simulink model "Frequency_scanning_2024a"  (R2024a)
settings: Solver=FixedStepAuto  StartTime=0  StopTime=2  FixedStep=Ts  RelTol=1e-3
InitFcn:
  | load('myData.mat')
  | 
  | %% Define parameters
  | xi=0;
  | w = 2*pi*50;
  | ApparatusPowerFlow{2} = [-P,-Q,V0,xi,w];
  | 
  | %% Mode
  | ApparatusType{2} = 10;
values from neighbouring files (symbols this model uses):
  x_e = [i_d; i_q; i_d_i; i_q_i; v_d_i; v_q_i; theta; v_dc; v_dc_i; i; i_i; v_lk; p_sum_i; p_lk_i]    [InterlinkAcDcB2B.m]
undefined symbols (not defined in the file or in its folder): ApparatusDiscreDamping, ApparatusPara, ApparatusPowerFlow, ApparatusType, cycles_n, DiscIntNeverNeededParam, f_end, f_start, harmonics_deg, n_sample, OtherInputs, PowerFlow, settle_time, start_time, submag, supmag, Ts, Vbase, Wbase, Zbase
libraries: SimplusGT x4, spsGroundLib x3, simulink x3, spsControlledVoltageSourceLib x3, spsVoltageMeasurementLib x1, spsThreePhaseSeriesRLCBranchLib x1, spspowerguiLib x1
settings Model: Creator=Yuming  LastModifiedBy=Yuming
settings DataIOCC: SaveOutput=off  SignalLogging=off  DSMLogging=off  InspectSignalLogs=on  SaveTime=off  ReturnWorkspaceOutputs=off
settings ConfigComp: CovBoundaryAbsTol=1.0e-5

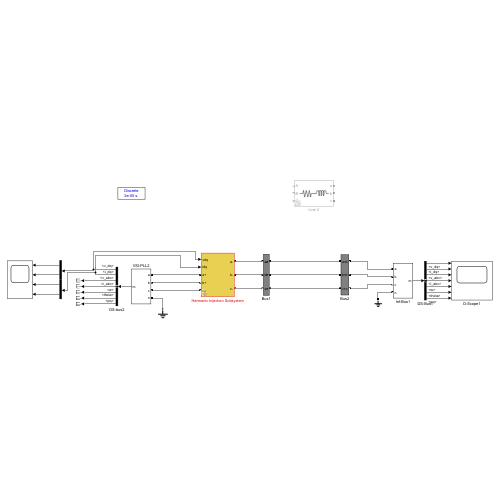
[thumbnail: Simulink's stored preview of the top-level diagram]
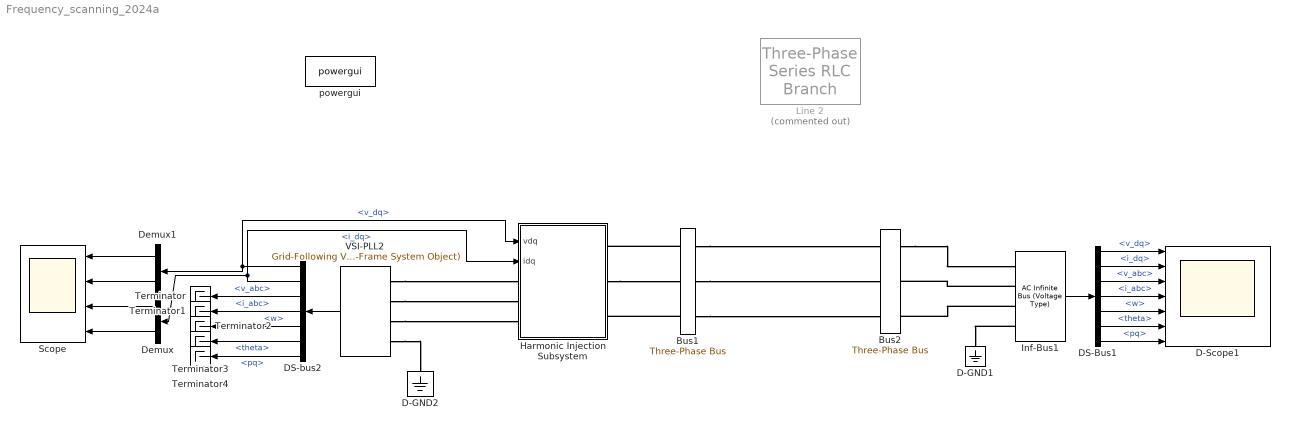
== system Frequency_scanning_2024a ==
  Bus1 : SimplusGT/Three-Phase Bus  Vbase=1  Sbase=1
      settings: SourceProductName=Simplus Grid Tool
  Bus2 : SimplusGT/Three-Phase Bus  Vbase=1  Sbase=1
      settings: SourceProductName=Simplus Grid Tool
  D-GND1 : spsGroundLib/Ground  LConnTagsString=a
  D-GND2 : spsGroundLib/Ground  LConnTagsString=a
  D-Scope1 : Scope  NumInputPorts=7
  DS-Bus1 : BusSelector  OutputSignals=v_dq,i_dq,v_abc,i_abc,w,theta,pq
  DS-bus2 : BusSelector  OutputSignals=v_dq,i_dq,v_abc,i_abc,w,theta,pq
  Demux : Demux  Outputs=2
  Demux1 : Demux  Outputs=2
  Harmonic Injection Subsystem : Subsystem  mask{f_start=f_start, f_end=f_end, n_pts=n_sample, cycle_collected=cycles_n, fundal_freq=50, start_time=start_time, settling_time=settle_time, subsyc_mag=submag, supsyc_mag=supmag, initial_phase=0, phase_angle=harmonics_deg}
      mask prompts: f_start "Start frequency (Hz)"; f_end "End frequency (Hz)"; n_pts "Number of samples"; cycle_collected "Full cycles in window"; fundal_freq "Fundamental Frequency (Hz)"; start_time "Start Time (sec)"; settling_time "Pre-settling duration (sec)"; subsyc_mag "Sub-synchronous magnitude (pu)"; supsyc_mag "Super-synchronous magnitude (pu)"; initial_phase "Initial phase (rad)"; phase_angle "Initial phase angle (w.r.t. fundamental) [deg]"
      mask init:
      | % Mask Initialization Code
      | freq_list = logspace(log10(f_start), log10(f_end), n_pts).';
      | idx_list  = (1:n_pts).';
      mask DialogControl DescGroupVar Prompt: Harmonic signal generator
      mask DialogControl DescTextVar Prompt: This block implements a harmonic signal generator.   It produces a fundamental component at the specified fundamental frequency,   together with two symmetrical sidebands (sub-synchronous and super-synchronous)   around the fundamental.
  Inf-Bus1 : SimplusGT/AC Infinite Bus (Voltage Type)  Ts=Ts  Sbase=Sbase  Vbase=Vbase  Wbase=Wbase  vd=PowerFlow{1}(3)  vq=0  theta0=PowerFlow{1}(4)  w=Wbase  R=1e-30
      settings: SourceProductName=Simplus Grid Tool
  Line 2 : spsThreePhaseSeriesRLCBranchLib/Three-Phase Series RLC Branch  Commented=on  LConnTagsString=A|B|C  RConnTagsString=A|B|C  BranchType=RL  Resistance=0.06*Zbase  Inductance=0.3*Zbase/Wbase  Capacitance=1e-6  Measurements=None
  Scope : Scope  NumInputPorts=4
  Terminator{,1..4} (5 alike) : Terminator
  VSI-PLL2 : SimplusGT/Grid-Following Voltage-Source Inverter (dq-Frame System Object)  Ts=Ts  Sbase=Sbase  Vbase=Vbase  Wbase=Wbase  ApparatusType=ApparatusType{2}  ApparatusPara=ApparatusPara{2}  PowerFlow=ApparatusPowerFlow{2}  x0=x_e{2}  OtherInputs=OtherInputs{2}  DiscreMethod=Hybrid Trapezoidal  EnableInsideModification=off  DiscreDampingFlag=on  DiscreDampingValue=ApparatusDiscreDamping{2}  LinearizationTimes=1  DirectFeedthrough=off
      settings: SourceProductName=Simplus Grid Tool
  powergui : spspowerguiLib/powergui  Priority=1  SimulationMode=Discrete  SampleTime=Ts  frequency=60  Iterations=50  frequencyindice=0  Pbase=100e6  ErrMax=1e-4  UnitsV=kV  UnitsW=MW  buscounter=0  FunctionMessages=off  echomessages=off  EnableUseOfTLC=off  CurrentSourceSwitches=off  DisableSnubberDevices=off  DisableRonSwitches=off  DisableVfSwitches=off  DisplayEquations=off  AutomaticDiscreteSolvers=off  SolverType=Tustin/Backward Euler (TBE)  Interpol=off  ExternalGateDelay=off  methode=off  Ts=100  x0status=blocks  SPID=on  SwTol=0  HookPort=off  NonlinearTolerance=1e-4  nMaxIteration=100  ContinueOnMaxIteration=off  RestoreLinks=warning  ResistiveCurrentMeasurement=off  Frange=[0:2:500]  Ylog=off  Xlog=on  ShowGrid=off  save=off  variable=ZData  structure=0  ZoomFFT=off  StartTime=0.0  cycles=1  DisplayStyle=1  fundamental=60  FreqAxis=off  MaxFrequency=1000  frequencyindicesteady=1  RmsSteady=1  display=off
  wires:
  Inf-Bus1/1 -> DS-Bus1/1
  DS-Bus1/1 -> D-Scope1/1  "<v_dq>"
  DS-Bus1/2 -> D-Scope1/2  "<i_dq>"
  DS-Bus1/3 -> D-Scope1/3  "<v_abc>"
  DS-Bus1/4 -> D-Scope1/4  "<i_abc>"
  DS-Bus1/5 -> D-Scope1/5  "<w>"
  DS-Bus1/6 -> D-Scope1/6  "<theta>"
  DS-Bus1/7 -> D-Scope1/7  "<pq>"
  VSI-PLL2/1 -> DS-bus2/1
  DS-bus2/1 -> Demux1/1, Harmonic Injection Subsystem/1(vdq)  "<v_dq>"
  DS-bus2/2 -> Demux/1, Harmonic Injection Subsystem/2(idq)  "<i_dq>"
  DS-bus2/3 -> Terminator/1  "<v_abc>"
  DS-bus2/4 -> Terminator1/1  "<i_abc>"
  DS-bus2/5 -> Terminator2/1  "<w>"
  DS-bus2/6 -> Terminator3/1  "<theta>"
  DS-bus2/7 -> Terminator4/1  "<pq>"
  Demux1/1 -> Scope/1
  Demux1/2 -> Scope/2
  Demux/1 -> Scope/3
  Demux/2 -> Scope/4
  connections:
  Inf-Bus1/LConn4 -- D-GND1/LConn1
  VSI-PLL2/LConn4 -- D-GND2/LConn1
  Inf-Bus1/LConn2 -- Bus2/RConn2
  Inf-Bus1/LConn3 -- Bus2/RConn3
  Bus1/RConn2 -- Bus2/LConn2
  Bus1/RConn1 -- Bus2/LConn1
  Bus1/RConn3 -- Bus2/LConn3
  Bus2/RConn1 -- Inf-Bus1/LConn1
  Bus1/LConn1 -- Harmonic Injection Subsystem/RConn1
  Harmonic Injection Subsystem/RConn2 -- Bus1/LConn2
  Bus1/LConn3 -- Harmonic Injection Subsystem/RConn3
  VSI-PLL2/LConn1 -- Harmonic Injection Subsystem/LConn1
  VSI-PLL2/LConn2 -- Harmonic Injection Subsystem/LConn2
  VSI-PLL2/LConn3 -- Harmonic Injection Subsystem/LConn3

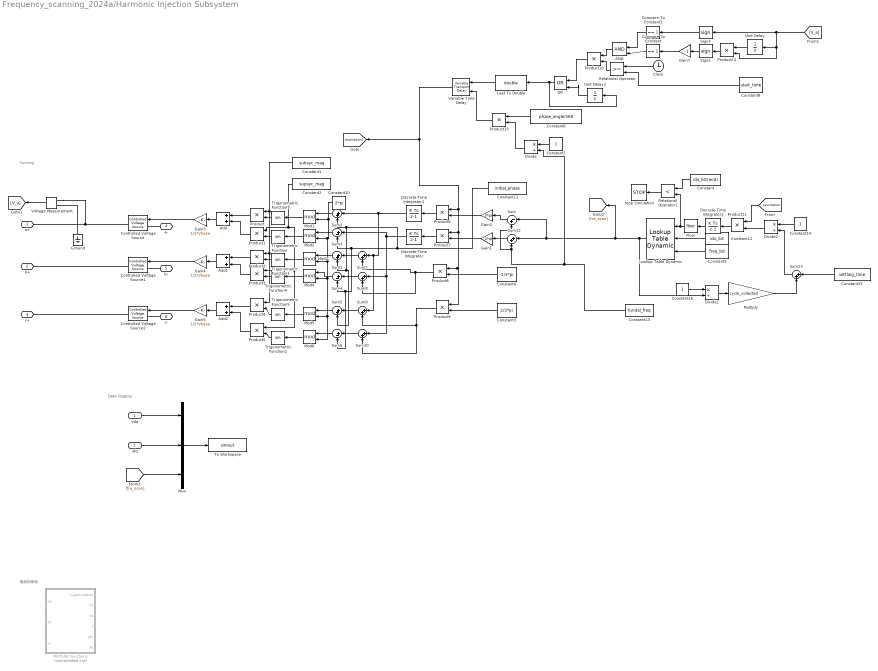
== system Frequency_scanning_2024a/Harmonic Injection Subsystem ==
  note: Data logging
  note: Yuming
  note: 废品回收站
  vdq : Inport
  idq : Inport  Port=2
  AND : Logic  IconShape=distinctive  AllPortsSameDT=off  OutDataTypeStr=boolean
  Add : Sum
  Add1 : Sum
  Add2 : Sum
  Cast To Double : DataTypeConversion  OutDataTypeStr=double  SaturateOnIntegerOverflow=off  RndMeth=Floor
  Clock : Clock
  Compare To Constant : simulink/Logic and Bit Operations/Compare To Constant  relop===  const=1  OutDataTypeStr=boolean
  Compare To Constant1 : simulink/Logic and Bit Operations/Compare To Constant  relop===  const=1  OutDataTypeStr=boolean
  Constant : Constant  Value=idx_list(end)
  Constant1 : Constant  Value=subsyc_mag
  Constant10 : Constant  Value=2*pi
  Constant11 : Constant  Value=initial_phase
  Constant12 : Constant  Value=idx_list
  Constant13 : Constant  Value=fundal_freq
  Constant14 : Constant
  Constant15 : Constant  Value=settling_time
  Constant16 : Constant
  Constant2 : Constant  Value=supsyc_mag
  Constant3 : Constant  Value=2/3*pi
  Constant4 : Constant  Value=-2/3*pi
  Constant5 : Constant  Value=freq_list
  Constant6 : Constant  Value=phase_angle/360
  Constant7 : Constant
  Constant9 : Constant  Value=start_time
  Controlled Voltage Source : spsControlledVoltageSourceLib/Controlled Voltage Source  Initialize=on  Source_Type=AC  Amplitude=0  Phase=0  Frequency=0  Measurements=None
  Controlled Voltage Source1 : spsControlledVoltageSourceLib/Controlled Voltage Source  Initialize=on  Source_Type=AC  Amplitude=0  Phase=0  Frequency=0  Measurements=None
  Controlled Voltage Source2 : spsControlledVoltageSourceLib/Controlled Voltage Source  Initialize=on  Source_Type=AC  Amplitude=0  Phase=0  Frequency=0  Measurements=None
  Discrete-Time Integrator : DiscreteIntegrator  SampleTime=Ts  ICPrevOutput=DiscIntNeverNeededParam  ICPrevScaledInput=DiscIntNeverNeededParam
  Discrete-Time Integrator1 : DiscreteIntegrator  SampleTime=Ts  ICPrevOutput=DiscIntNeverNeededParam  ICPrevScaledInput=DiscIntNeverNeededParam
  Discrete-Time Integrator2 : DiscreteIntegrator  SampleTime=-1  ICPrevOutput=DiscIntNeverNeededParam  ICPrevScaledInput=DiscIntNeverNeededParam
  Divide : Product  Inputs=*/
  Divide1 : Product  Inputs=*/
  Divide2 : Product  Inputs=*/
  Floor : Rounding
  Gain1 : Gain  Gain=2*pi
  Gain2 : Gain  Gain=2*pi
  Gain3 : Gain  Gain=1/2*Vbase
  Gain4 : Gain  Gain=1/2*Vbase
  Gain5 : Gain  Gain=1/2*Vbase
  Gain7 : Gain  Gain=-1
  Ground : spsGroundLib/Ground  LConnTagsString=a
  Lookup Table Dynamic : simulink/Lookup Tables/Lookup Table Dynamic  LookUpMeth=Interpolation-Use End Values  OutDataType=fixdt('double')  OutScaling=[]  OutputDataTypeScalingMode=Specify via dialog  OutDataTypeStr=double  DoSatur=off
  MATLAB Function1 : MATLAB Function  Commented=on  TreatAsAtomicUnit=on
  Mod{1..6} (6 alike) : Math  Operator=mod
  Multiply : Gain  Gain=cycle_collected
  Mux : Mux  Inputs=3
  OR : Logic  Operator=OR  IconShape=distinctive  AllPortsSameDT=off  OutDataTypeStr=boolean
  Product{,1..13} (14 alike) : Product
  Relational Operator : RelationalOperator  OutDataTypeStr=boolean  RndMeth=Simplest  InputSameDT=off
  Relational Operator1 : RelationalOperator  Operator=<  OutDataTypeStr=boolean  RndMeth=Simplest  InputSameDT=off
  Sign2 : Signum
  Sign3 : Signum
  Stop Simulation : Stop
  Sum : Sum  Inputs=|-+
  Sum{1..2,5,7..10,12..13} (9 alike) : Sum  Inputs=|++
  Sum3 : Sum  Inputs=|+-
  Sum4 : Sum  Inputs=|+-
  Sum6 : Sum  Inputs=|+-
  To Workspace : ToWorkspace  VariableName=simout  SaveFormat=Timeseries  SampleTime=-1
  Trigonometric Function{,1..5} (6 alike) : Trigonometry
  Unit Delay : UnitDelay  SampleTime=-1  HasFrameUpgradeWarning=on
  Unit Delay2 : UnitDelay  SampleTime=-1  HasFrameUpgradeWarning=on
  Variable Time Delay : VariableTransportDelay  MaximumDelay=10
  Voltage Measurement : spsVoltageMeasurementLib/Voltage Measurement  PhasorSimulation=off  OutputType=Complex  PSBequivalent=0
  a+ : PMIOPort  Side=Left
  b+ : PMIOPort  Port=2  Side=Left
  c+ : PMIOPort  Port=3  Side=Left
  a- : PMIOPort  Port=4  Side=Right
  b- : PMIOPort  Port=5  Side=Right
  c- : PMIOPort  Port=6  Side=Right
  wires:
  Constant1/1 -> Product4/1, Product2/1, Product/1
  Constant2/1 -> Product5/1, Product3/1, Product1/1
  Constant11/1 -> Sum6/2, Sum4/2, Sum3/2, Sum5/2, Sum1/2, Sum2/2
  Add/1 -> Gain3/1
  Add1/1 -> Gain4/1
  Add2/1 -> Gain5/1
  Trigonometric Function3/1 -> Product/2
  Product/1 -> Add/1
  Trigonometric Function/1 -> Product1/2
  Product1/1 -> Add/2
  Product2/1 -> Add1/1
  Trigonometric Function1/1 -> Product2/2
  Trigonometric Function4/1 -> Product3/2
  Trigonometric Function2/1 -> Product5/2
  Trigonometric Function5/1 -> Product4/2
  Product4/1 -> Add2/1
  Product5/1 -> Add2/2
  Discrete-Time Integrator1/1 -> Sum7/1, Sum9/1, Sum2/1
  Discrete-Time Integrator/1 -> Sum8/1, Sum10/1, Sum3/1
  Sum7/1 -> Sum1/1
  Sum8/1 -> Sum4/1
  Sum9/1 -> Sum5/1
  Sum10/1 -> Sum6/1
  Sum/1 -> Gain2/1
  Sum12/1 -> Gain1/1
  Lookup Table Dynamic/1 -> Divide1/2, [fre_scan], Sum/1, Sum12/1
  Product3/1 -> Add1/2
  Mod1/1 -> Trigonometric Function3/1
  Mod2/1 -> Trigonometric Function/1
  Mod3/1 -> Trigonometric Function1/1
  Mod4/1 -> Trigonometric Function4/1
  Mod6/1 -> Trigonometric Function2/1
  Mod5/1 -> Trigonometric Function5/1
  Sum2/1 -> Mod1/1
  Sum3/1 -> Mod2/1
  Sum1/1 -> Mod3/1
  Sum4/1 -> Mod4/1
  Sum5/1 -> Mod5/1
  Sum6/1 -> Mod6/1
  Constant10/1 -> Mod6/2, Mod5/2, Mod4/2, Mod3/2, Mod2/2, Mod1/2
  Gain3/1 -> Controlled Voltage Source/1
  Gain4/1 -> Controlled Voltage Source1/1
  Gain5/1 -> Controlled Voltage Source2/1
  Product6/1 -> Discrete-Time Integrator1/1
  Product7/1 -> Discrete-Time Integrator/1
  Constant3/1 -> Product9/2
  Constant4/1 -> Product8/2
  Gain1/1 -> Product7/2
  Gain2/1 -> Product6/2
  Product8/1 -> Sum7/2, Sum8/2
  Product9/1 -> Sum9/2, Sum10/2
  Constant5/1 -> Lookup Table Dynamic/3
  Constant12/1 -> Lookup Table Dynamic/2
  Discrete-Time Integrator2/1 -> Floor/1
  Divide2/1 -> Product11/2
  Product11/1 -> Discrete-Time Integrator2/1
  [excitation] -> Product11/1
  Relational Operator1/1 -> Stop Simulation/1
  Constant/1 -> Relational Operator1/1
  Constant16/1 -> Divide1/1
  Divide1/1 -> Multiply/1
  Constant15/1 -> Sum13/1
  Multiply/1 -> Sum13/2
  Sum13/1 -> Divide2/2
  Constant14/1 -> Divide2/1
  Floor/1 -> Relational Operator1/2, Lookup Table Dynamic/1
  Voltage Measurement/1 -> [V_a]
  idq/1 -> Mux/2
  vdq/1 -> Mux/1
  [fre_scan] -> Mux/3
  Mux/1 -> To Workspace/1
  Variable Time Delay/1 -> Product8/1, Product9/1, Product7/1, Product6/1, [excitation]
  Constant7/1 -> Divide/1
  OR/1 -> Unit Delay2/1, Cast To Double/1
  Constant9/1 -> Relational Operator/2
  Clock/1 -> Relational Operator/1
  Divide/1 -> Product13/2
  Sign3/1 -> Compare To Constant1/1
  Constant13/1 -> Divide/2, Sum/2, Sum12/2
  [V_a] -> Product12/2, Unit Delay/1, Sign3/1
  Cast To Double/1 -> Variable Time Delay/1
  Constant6/1 -> Product13/1
  Sign2/1 -> Gain7/1
  Product12/1 -> Sign2/1
  Compare To Constant/1 -> AND/2
  Product10/1 -> OR/1
  Relational Operator/1 -> Product10/2
  AND/1 -> Product10/1
  Product13/1 -> Variable Time Delay/2
  Unit Delay2/1 -> OR/2
  Compare To Constant1/1 -> AND/1
  Gain7/1 -> Compare To Constant/1
  Unit Delay/1 -> Product12/1
  connections:
  a-/RConn1 -- Controlled Voltage Source/LConn1
  c-/RConn1 -- Controlled Voltage Source2/LConn1
  b-/RConn1 -- Controlled Voltage Source1/LConn1
  Controlled Voltage Source/RConn1 -- Voltage Measurement/LConn1 -- a+/RConn1
  Controlled Voltage Source1/RConn1 -- b+/RConn1
  Controlled Voltage Source2/RConn1 -- c+/RConn1
  Ground/LConn1 -- Voltage Measurement/LConn2

== matlab function Frequency_scanning_2024a/Harmonic Injection Subsystem/MATLAB Function1 ==
  data: f_perturbation input; va output; Vs input; Vc input; t input; phi input; vb output; vc output; f0 input
function [va, vb, vc] = fcn(f_perturbation, Vs, Vc, t, phi,f0)
% Harmonic Injection Subsystem (three-phase, 50 Hz-centered sidebands)
%
% Inputs:
%   f_delta [Hz] : Frequency offset from 50 Hz, i.e. sidebands at 50+Δf and 50−Δf
%   Vs     [V]   : Amplitude of the upper sideband (50+Δf)
%   Vc     [V]   : Amplitude of the lower sideband (50−Δf)
%   t      [s]   : Current simulation time (connect from Simulink Clock block)
%   phi    [rad] : Phase offset (set to 0 if not needed)
%
% Outputs:
%   va,vb,vc: Three-phase injected signals, phase-shifted by 120°

% ---- guards ----
if nargin < 6 || f0 <= 0
    f0 = 50; % fallback
end
f = max(f_perturbation, 0); % non-negative frequency

% Mirror the given absolute frequency around f0 to form symmetric pair
if f >= f0
    f_up   = f;
    f_down = max(2*f0 - f, 1e-6); % keep > 0
    phi_u = phi;  % upper sideband
    phi_d = -phi;  % lower sideband
else
    f_down = max(f, 1e-6);
    f_up   = 2*f0 - f;
    phi_u = -phi;  % upper sideband
    phi_d = phi;  % lower sideband
end

% Phase angles for the two components
th_up   = 2*pi*f_up*t + phi_u;
th_down = 2*pi*f_down*t + phi_d;

% Phase shift for each phase (abc, 120° apart)
phi_a = 0;
phi_b = -2*pi/3;   % -120°
phi_c =  2*pi/3;   % +120°

% Generate three-phase signals (sum of upper and lower sidebands)
va = Vc*sin(th_up   + phi_a) + Vs*sin(th_down + phi_a);
vb = Vc*sin(th_up   + phi_b) + Vs*sin(th_down + phi_b);
vc = Vc*sin(th_up   + phi_c) + Vs*sin(th_down + phi_c);
end
